simulink model "modemodemodel"  (R2020a)
settings: Solver=ode8  StartTime=0.0  StopTime=5  FixedStep=0.002  RelTol=1e-3
InitFcn:
  | Ao=(0.70*0.001)^2*pi/4;
  | 
  | 
  | 
  | Ar=0.38*10^-6;
  | Aor=0.1*10^-6;
  | Ap=(32.50*0.001)^2*pi/4;
  | 
  | kappaaa=1.4-1.4*(Aor/Ap);
  | 
  | kappa=1.4;
  | x0=0.042;
  | P0=101325;
  | row0=1.1841;
  | T=0.005;
  | Cor=0.8;
  | 
  | Fmax=15;
  | Xmax=0.004;
  | Vmax=0.1;
  | B=0;
libraries: simulink x2
settings Model: Creator=hiratsuka  LastModifiedBy=Peanatsu
settings DataIOCC: ReturnWorkspaceOutputs=off
settings DebuggingCC: ArithmeticOperatorsInVariantConditions=warning
settings SFSimCC: SimUseLocalCustomCode=off  CustomCodeUndefinedFunction=UseInterfaceOnly
settings RTWCC: RTWUseLocalCustomCode=off

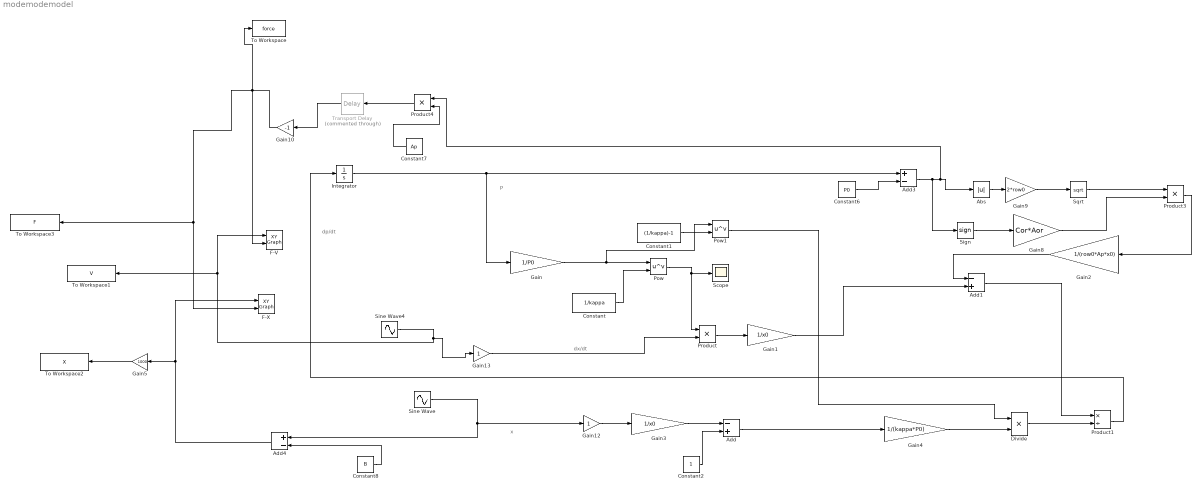
== system modemodemodel ==
  note: dx/dt
  note: x
  note: P
  note: dp/dt
  Abs : Abs
  Add : Sum  Inputs=-+
  Add1 : Sum  Inputs=-+
  Add3 : Sum  Inputs=+-
  Add4 : Sum  Inputs=+-
  Constant : Constant  Value=1/kappa
  Constant1 : Constant  Value=(1/kappa)-1
  Constant2 : Constant
  Constant6 : Constant  Value=P0
  Constant7 : Constant  Value=Ap
  Constant8 : Constant  Value=B
  Divide : Product  Inputs=**
  F-V : simulink/Sinks/XY Graph  xmin=-Vmax  xmax=Vmax  ymin=-Fmax  ymax=Fmax  st=-1
  F-X : simulink/Sinks/XY Graph  xmin=-Xmax  xmax=Xmax  ymin=-Fmax  ymax=Fmax  st=-1
  Gain : Gain  Gain=1/P0
  Gain1 : Gain  Gain=1/x0
  Gain10 : Gain  Gain=-1
  Gain12 : Gain
  Gain13 : Gain
  Gain2 : Gain  Gain=1/(row0*Ap*x0)
  Gain3 : Gain  Gain=1/x0
  Gain4 : Gain  Gain=1/(kappa*P0)
  Gain5 : Gain  Gain=1000
  Gain8 : Gain  Gain=Cor*Aor
  Gain9 : Gain  Gain=2*row0
  Integrator : Integrator  InitialCondition=101325
  Pow : Math  Operator=pow  SignedPower=on  OutputSignalType=real  RndMeth=Zero  SaturateOnIntegerOverflow=on
  Pow1 : Math  Operator=pow  SignedPower=on  OutputSignalType=real  RndMeth=Zero  SaturateOnIntegerOverflow=on
  Product : Product
  Product1 : Product  Inputs=*/
  Product3 : Product
  Product4 : Product
  Scope : Scope
  Sign : Signum
  Sine Wave : Sin  Amplitude=0.003  Bias=B  Frequency=2*pi*5  SampleTime=0
  Sine Wave4 : Sin  Amplitude=0.003*2*pi*5  Bias=B  Frequency=2*pi*5  Phase=pi/2  SampleTime=0
  Sqrt : Sqrt  SaturateOnIntegerOverflow=on
  To Workspace : ToWorkspace  VariableName=force  SampleTime=-1
  To Workspace1 : ToWorkspace  VariableName=V  SaveFormat=Timeseries  SampleTime=-1
  To Workspace2 : ToWorkspace  VariableName=X  SaveFormat=Timeseries  SampleTime=-1
  To Workspace3 : ToWorkspace  VariableName=F  SaveFormat=Timeseries  SampleTime=-1
  Transport Delay : TransportDelay  Commented=through  DelayTime=0
  wires:
  Constant/1 -> Pow/2
  Gain/1 -> Pow1/1, Pow/1
  Pow/1 -> Scope/1, Product/1
  Product/1 -> Gain1/1
  Constant1/1 -> Pow1/2
  Gain3/1 -> Add/1
  Constant2/1 -> Add/2
  Add/1 -> Gain4/1
  Gain4/1 -> Divide/2
  Pow1/1 -> Divide/1
  Divide/1 -> Product1/2
  Product1/1 -> Integrator/1
  Sign/1 -> Gain8/1
  Constant6/1 -> Add3/2
  Integrator/1 -> Gain/1, Add3/1
  Gain8/1 -> Product3/2
  Product3/1 -> Gain2/1
  Add1/1 -> Product1/1
  Abs/1 -> Gain9/1
  Constant7/1 -> Product4/2
  Constant8/1 -> Add4/2
  Gain9/1 -> Sqrt/1
  Sine Wave/1 -> Gain12/1, Add4/1
  Gain12/1 -> Gain3/1
  Sine Wave4/1 -> Gain13/1, To Workspace1/1, F-V/1
  Gain2/1 -> Add1/1
  Gain13/1 -> Product/2
  Gain1/1 -> Add1/2
  Sqrt/1 -> Product3/1
  Add3/1 -> Sign/1, Product4/1, Abs/1
  Product4/1 -> Transport Delay/1
  Transport Delay/1 -> Gain10/1
  Gain10/1 -> F-V/2, F-X/2, To Workspace3/1, To Workspace/1
  Add4/1 -> F-X/1, Gain5/1
  Gain5/1 -> To Workspace2/1
